simulink model "Robot3_CL2"  (R2021a)
settings: Solver=ode4  StartTime=0.0  StopTime=10.0  RelTol=1e-3
undefined symbols (not defined in the file): sigbuilder_block
settings Model: Creator=Patel  LastModifiedBy=Patel

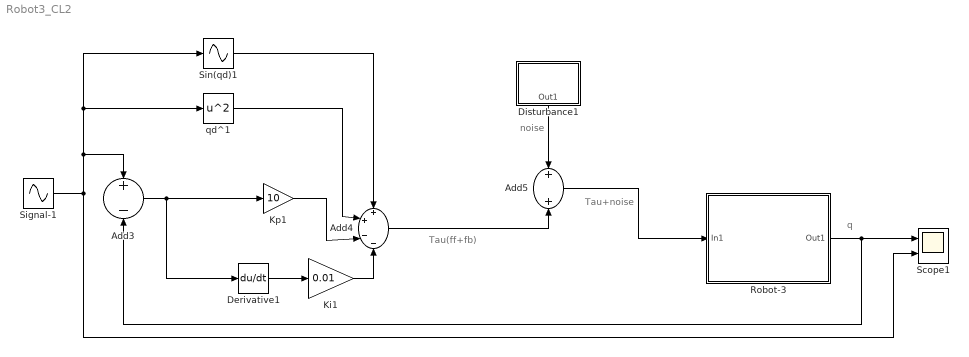
== system Robot3_CL2 ==
  note: q
  note: Tau+noise
  note: noise
  note: Tau(ff+fb)
  Add3 : Sum  Inputs=+-
  Add4 : Sum  Inputs=++--
  Add5 : Sum
  Derivative1 : Derivative
  Disturbance1 : Subsystem
  Ki1 : Gain  Gain=0.01
  Kp1 : Gain  Gain=10
  Robot-3 : Subsystem
  Scope1 : Scope  NumInputPorts=2
  Signal-1 : Sin  Frequency=2*pi*1  SampleTime=0
  Sin(qd)1 : Sin  TimeSource=Use external signal  SampleTime=0
  qd^1 : Math  Operator=square  SaturateOnIntegerOverflow=on
  wires:
  Add4/1 -> Add5/2
  Signal-1/1 -> Sin(qd)1/1, qd^1/1, Add3/1, Scope1/2
  Add5/1 -> Robot-3/1(In1)
  Robot-3/1(Out1) -> Scope1/1, Add3/2
  Ki1/1 -> Add4/4
  Kp1/1 -> Add4/3
  Add3/1 -> Derivative1/1, Kp1/1
  Disturbance1/1(Out1) -> Add5/1
  qd^1/1 -> Add4/2
  Derivative1/1 -> Ki1/1
  Sin(qd)1/1 -> Add4/1

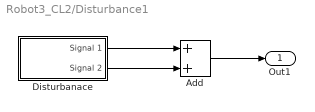
== system Robot3_CL2/Disturbance1 ==
  Add : Sum
  Disturbanace : Subsystem  Tag=STV Subsys  LoadFcn=sigbuilder_block('load');  StartFcn=sigbuilder_block('start');  StopFcn=sigbuilder_block('stop');  ClipboardFcn=sigbuilder_block('clipboard');  mask(Sigbuilder block){tuvar=[0:10]}
      mask help: Simulink:masks:SigbuilderBlock_MD
      mask init:
      | if ~strcmp(get_param(bdroot(gcbh),'SimulationStatus'),'stopped') tuvar = sigbuilder_block('maskInit'); end
      settings: CopyFcn=sigbuilder_block('copy');  DeleteFcn=sigbuilder_block('delete');  ModelCloseFcn=sigbuilder_block('modelClose');  PreSaveFcn=sigbuilder_block('preSave');  PauseFcn=sigbuilder_block('pause');  ContinueFcn=sigbuilder_block('continue');  NameChangeFcn=sigbuilder_block('namechange');  OpenFcn=sigbuilder_block('open',[437.6 153 550.4 359.25 ]);  CloseFcn=sigbuilder_block('close');
      mask Display: plot(0, 0, 100, 100,[2, 2, 32, 32, 2], [68, 8, 8, 68, 68],[32, 2], [38, 38], [32, 19, 2],[53, 60, 44], [32, 17, 17, 2],[16, 16, 31, 31]);txt = getActiveGroup(gcbh);text(2, 100, txt,'verticalAlignment', 'top');
  Out1 : Outport
  wires:
  Disturbanace/1(Signal 1) -> Add/1
  Disturbanace/2(Signal 2) -> Add/2
  Add/1 -> Out1/1

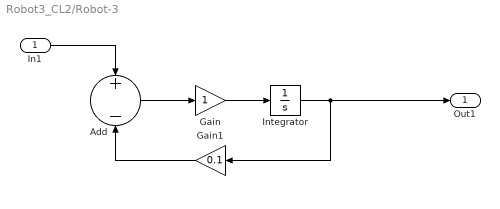
== system Robot3_CL2/Robot-3 ==
  In1 : Inport
  Add : Sum  Inputs=+-
  Gain : Gain
  Gain1 : Gain  Gain=0.1
  Integrator : Integrator
  Out1 : Outport
  wires:
  Integrator/1 -> Gain1/1, Out1/1
  In1/1 -> Add/1
  Gain/1 -> Integrator/1
  Gain1/1 -> Add/2
  Add/1 -> Gain/1

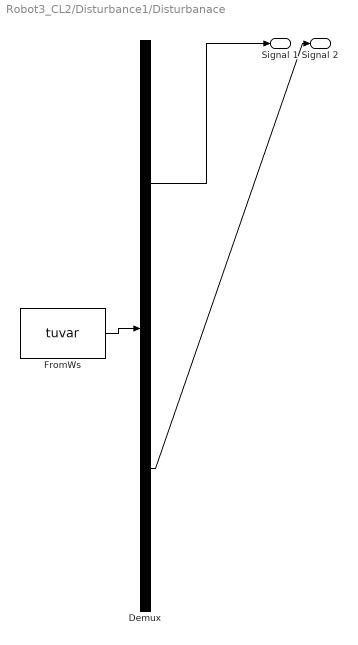
== system Robot3_CL2/Disturbance1/Disturbanace ==
  Demux : Demux  Tag=STV Demux  Outputs=2
      settings: DisplayOption=none
  FromWs : FromWorkspace  Tag=STV FromWs  VariableName=tuvar
      SigBuilderData=|
      | common.afterFinalStr = 'Extrapolate'
      | common.sampleTime = 0
      | dataSet.timeRange = [0 10]
      | dataSet.name = 'Group 1'
      | sbobj.Groups.Name = 'Group 1'
      | sbobj.Groups.Signals(1).Name = 'Signal 1'
      | sbobj.Groups.Signals(1).XData = [0 0.1 0.2 0.3 0.4 0.5 0.6 0.7 0.8 0.9 1 1.1 1.2 1.3 1.4 1.5 1.6 1.7 1.8 1.9 2 2.1 2.2 2.3 2.4 2.5 2.6 2.7 2.8 2.9 3 3.1 3.2 3.3 3.4 3.5 3.6 3.7 3.8 3.9 4 4.1 4.2 4.3 4.4 4.5 4.6 4.7 4.8 4.9 5 5.1 5.2 5.3 5.4 5.5 5.6 5.7 5.8 5.9 6 6.1 6.2 6.3 6.4 6.5 6.6 6.7 6.8 6.9 7 7.1 7.2 7.3 7.4 7.5 7.6 7.7 7.8 7.9 8 8.1 8.2 8.3 8.4 8.5 8.6 8.7 8.8 8.9 9 9.1 9.2 9.3 9.4 9.5 9.6 9.7 9.8 9.9 10]
      | sbobj.Groups.Signals(1).YData = [0.537667139546 1.8338850146 -2.258846861 0.862173320368 0.318765239859 -1.30768829631 -0.433592022306 0.342624466539 3.57839693973 2.76943702988 -1.34988694016 3.03492346633 0.725404224946 -0.0630548731897 0.714742903826 -0.2049660583 -0.124144348216 1.48969760779 1.4090344898 1.41719241343 0.671497133608 -1.20748692269 0.717238651329 1.63023528916 0.488893770312 1.03469300992 0.726885133383 -0.303440924786 0.293871467097 -0.787282803759 0.888395631758 -1.14707010697 -1.06887045817 -0.809498694425 -2.94428416199 1.43838029282 0.325190539456 -0.75492831917 1.3702985401 -1.71151641885 -0.102242446085 -0.241447041607 0.319206739166 0.312858596637 -0.864879917324 -0.0300512961963 -0.164879019209 0.627707287529 1.09326566904 1.10927329761 -0.863652821989 0.0773590911304 -1.21411704362 -1.11350074149 -0.00684932810335 1.53263030828 -0.769665913754 0.37137881276 -0.225584402271 1.11735613881 -1.08906429505 0.032557464165 0.552527021112 1.10061021788 1.5442118955 0.0859311331754 -1.49159031064 -0.74230183726 -1.06158173332 2.350457224 -0.615601881467 0.748076783704 -0.192418510588 0.888610425421 -0.764849236568 -1.40226896934 -1.42237592509 0.48819390986 -0.177375156619 -0.196053487807 1.41931015064 0.291584373984 0.197811053464 1.58769908997 -0.80446595635 0.69662441585 0.835088165073 -0.243715140378 0.215670086404 -1.16584393148 -1.1479527789 0.104874716016 0.722254032225 2.58549125262 -0.666890670701 0.187331024579 -0.082494425371 -1.93302291785 -0.438966153935 -1.79467884146 0.840375529754]
      | sbobj.Groups.Signals(2).Name = 'Signal 2'
      | sbobj.Groups.Signals(2).XData = [0 10]
      | sbobj.Groups.Signals(2).YData = [0.98 0.98]
  Signal 1 : Outport  Tag=STV Outport
  Signal 2 : Outport  Tag=STV Outport  Port=2
  wires:
  Demux/1 -> Signal 1/1
  FromWs/1 -> Demux/1
  Demux/2 -> Signal 2/1
